simulink model "hebianna"  (Simulink 7.5)
settings: Solver=ode45  StartTime=0.0  StopTime=10.0  RelTol=1e-3
settings Model: Creator=My Laptop  LastModifiedBy=My Laptop

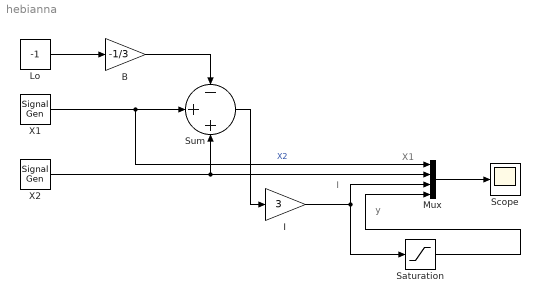
== system hebianna ==
  note: y
  note: I
  note: X1
  B : Gain  Gain=-1/3  ParameterDataType=fixdt(1, 16)  ParameterScaling=2^0  OutDataType=fixdt(1, 16)  OutScaling=2^0
  I : Gain  Gain=3  ParameterDataType=fixdt(1, 16)  ParameterScaling=2^0  OutDataType=fixdt(1, 16)  OutScaling=2^0
  Lo : Constant  Value=-1  OutDataType=fixdt(1, 16)  OutScaling=2^0
  Mux : Mux
  Saturation : Saturate  UpperLimit=1  LowerLimit=-1  ZeroCross=off  OutDataType=fixdt(1, 16)  OutScaling=2^0
  Scope : Scope
      settings: YMin=-8  YMax=8
  Sum : Sum  Inputs=-++  OutDataType=fixdt(1, 16)  OutScaling=2^0
  X1 : SignalGenerator  WaveForm=square  Frequency=.4
  X2 : SignalGenerator  WaveForm=square  Frequency=.2
  wires:
  Lo/1 -> B/1
  Mux/1 -> Scope/1
  B/1 -> Sum/1
  Sum/1 -> I/1
  X2/1 -> Mux/2, Sum/3
  I/1 -> Mux/3, Saturation/1
  X1/1 -> Sum/2, Mux/1  "X2"
  Saturation/1 -> Mux/4
